simulink model "EarlyReturn19_2018a"  (R2018a)
settings: Solver=VariableStepAuto  StartTime=0.0  StopTime=0.1  RelTol=1e-3
settings Model: Creator=BEAR  LastModifiedBy=apple

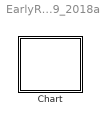
== system EarlyReturn19_2018a ==
  Chart : Stateflow chart  TreatAsAtomicUnit=on

== stateflow chart EarlyReturn19_2018a/Chart ==
  settings: updateMethod=DISCRETE  sampleTime=0.1
  state S
    en: fprintf("enS")
    du: fprintf("duS")
    ex: fprintf("exS")
    (junction 15) -> S : {fprintf("ca2")}/{fprintf("ta2")}
    S -> (junction 15) [order 1] : {fprintf("ca1")}/{E;fprintf("ta1")}
  state T
    en: fprintf("enT")
  (default) -> S
  S -> T [order 1] : E
  events: E local FUNCTION_CALL_EVENT
